simulink model "BatteryEstim3RC_PTBS_estimation"  (R2020b)
settings: Solver=ode45  StartTime=0.0  StopTime=runtime  FixedStep=stepSize  MaxStep=60  RelTol=1e-3
values from neighbouring files (symbols this model uses):
  Q = 277.758    [BatteryEstim3RC_run.m]
undefined symbols (not defined in the file or in its folder): coeff, init_Q, init_Vt, OCV_current, OCV_prev, R0_current, R0_prev, R1_current, R1_prev, R2_current, R2_prev, R3_current, R3_prev, SOC_current, SOC_prev, tau1_current, tau1_prev, tau2_current, tau2_prev, tau3_current, tau3_prev
libraries: autolibbatterycommon x4
settings Model: ModifiedByFormat=The MathWorks, Inc.  Creator=The MathWorks, Inc.  LastModifiedBy=The MathWorks, Inc.
settings DataIOCC: ExternalInput=[input_time input_current]  LoadExternalInput=on  SaveOutput=off  DSMLogging=off  SaveTime=off  ReturnWorkspaceOutputs=off
settings DebuggingCC: ArithmeticOperatorsInVariantConditions=warning
settings SFSimCC: SimUseLocalCustomCode=off  CustomCodeUndefinedFunction=UseInterfaceOnly
settings RTWCC: RTWUseLocalCustomCode=off
settings CodeAppCC: StateflowObjectComments=on

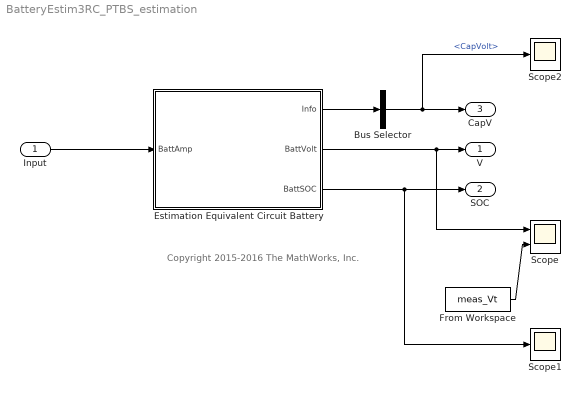
== system BatteryEstim3RC_PTBS_estimation ==
  note: Copyright 2015-2016 The MathWorks, Inc.
  Input : Inport
  Bus Selector : BusSelector  OutputSignals=CapVolt
  Estimation Equivalent Circuit Battery : Subsystem  mask(Estimation Equivalent Circuit Battery){NumRC=3, Em=[OCV_current; OCV_prev], R0=[R0_current; R0_prev], SOC_BP=[SOC_current; SOC_prev], BattCap=Q, BattCapInit=init_Q, InitialCapVoltage=init_Vt, R1=[R1_current; R1_prev], C1=[tau1_current./R1_current; tau1_prev./R1_prev], R2=[R2_current; R2_prev], C2=[tau2_current./R2_current; tau2_prev./R2_prev], R3=[R3_current; R3_prev], C3=[tau3_current./R3_current; tau3_prev./R3_prev], R4=[0.005 0.005 0.005 0.005 0.005 0.005], C4=[10000 10000 10000 10000 10000 10000], R5=[0.005 0.005 0.005 0.005 0.005 0.005], C5=[10000 10000 10000 10000 10000 10000], Vu=Inf, Vl=-Inf}
      mask prompts: NumRC "autoblks:autoblkParamEstRcBattery:blkPrm_NumRC"; Em "autoblks:autoblkParamEstRcBattery:blkPrm_Em"; R0 "autoblks:autoblkParamEstRcBattery:blkPrm_R0"; SOC_BP "autoblks:autoblkParamEstRcBattery:blkPrm_SOC_BP"; BattCap "autoblks:autoblkParamEstRcBattery:blkPrm_BattCap"; BattCapInit "autoblks:autoblkParamEstRcBattery:blkPrm_BattCapInit"; InitialCapVoltage "autoblks:autoblkParamEstRcBattery:blkPrm_InitialCapVoltage"; R1 "autoblks:autoblkParamEstRcBattery:blkPrm_R1"; C1 "autoblks:autoblkParamEstRcBattery:blkPrm_C1"; R2 "autoblks:autoblkParamEstRcBattery:blkPrm_R2"; C2 "autoblks:autoblkParamEstRcBattery:blkPrm_C2"; R3 "autoblks:autoblkParamEstRcBattery:blkPrm_R3"; C3 "autoblks:autoblkParamEstRcBattery:blkPrm_C3"; R4 "autoblks:autoblkParamEstRcBattery:blkPrm_R4"; C4 "autoblks:autoblkParamEstRcBattery:blkPrm_C4"; R5 "autoblks:autoblkParamEstRcBattery:blkPrm_R5"; C5 "autoblks:autoblkParamEstRcBattery:blkPrm_C5"; Vu "autoblks:autoblkParamEstRcBattery:blkPrm_Vu"; Vl "autoblks:autoblkParamEstRcBattery:blkPrm_Vl"
      mask help: autoblks:autoblkParamEstRcBattery:blkDesc
      mask init:
      | autoicon('pbbatteryparamest', gcb, 'Initialization');
      mask Help: eval('autoblkshelp(''pbbatteryrcnetworkpe'')');
      mask TypeOptions NumRC: autoblks:autoblkParamEstRcBattery:blkCmb_NumRC1 | autoblks:autoblkParamEstRcBattery:blkCmb_NumRC2 | autoblks:autoblkParamEstRcBattery:blkCmb_NumRC3 | autoblks:autoblkParamEstRcBattery:blkCmb_NumRC4 | autoblks:autoblkParamEstRcBattery:blkCmb_NumRC5
      mask Callback NumRC: autoicon('pbbatteryparamest', gcb, 'NumRCPopup');
      mask DialogControl Container9 Prompt: autoblks:autoblkParamEstRcBattery:blkDlg_Container9
      mask DialogControl NumRC Prompt: Number of series RC pairs:
      mask DialogControl Em Prompt: Open circuit voltage table data, Em [V]:
      mask DialogControl R0 Prompt: Series resistance table data, R0 [Ohm]:
      mask DialogControl SOC_BP Prompt: State of charge breakpoints, SOC_BP []:
      mask DialogControl BattCap Prompt: Battery capacity, BattCap [Ah]:
      mask DialogControl BattCapInit Prompt: Initial battery capacity, BattCapInit [Ah]:
      mask DialogControl InitialCapVoltage Prompt: Initial capacitor voltage, InitialCapVoltage [V]:
      mask DialogControl Container10 Prompt: autoblks:autoblkParamEstRcBattery:blkDlg_Container10
      mask DialogControl R1 Prompt: Network resistance table data, R1 [Ohm]:
      mask DialogControl C1 Prompt: Network capacitance table data, C1 [F]:
      mask DialogControl R2 Prompt: Network resistance table data, R2 [Ohm]:
      mask DialogControl C2 Prompt: Network capacitance table data, C2 [F]:
      mask DialogControl R3 Prompt: Network resistance table data, R3 [Ohm]:
      mask DialogControl C3 Prompt: Network capacitance table data, C3 [F]:
      mask DialogControl R4 Prompt: Network resistance table data, R4 [Ohm]:
      mask DialogControl C4 Prompt: Network capacitance table data, C4 [F]:
      mask DialogControl R5 Prompt: Network resistance table data, R5 [Ohm]:
      mask DialogControl C5 Prompt: Network capacitance table data, C5 [F]:
      mask DialogControl Container7 Prompt: autoblks:autoblkParamEstRcBattery:blkDlg_Container7
      mask DialogControl Vu Prompt: Upper Integrator Voltage Limit, Vu [V]:
      mask DialogControl Vl Prompt: Lower Integrator Voltage Limit, Vl [V]:
      mask Display:
      | IconInfo = autoicon('pbbatteryparamest', gcb, 'DrawCommands');
      | 
      | image(IconInfo.image, IconInfo.position);
      | 
      | for i = 1:numel(IconInfo.lconn)
      |     port_label('lconn', i, IconInfo.lconn{i})
      | end
      | 
      | for j = 1:numel(IconInfo.rconn)
      |     port_label('rconn', j, IconInfo.rconn{j})
      | end
      | 
      | for k = 1:numel(IconInfo.input)
      |     port_label('input', k, IconInfo.input{k})
      | end
      | 
      | for m = 1:numel(IconInfo.output)
      |     port_label('output', m, IconInfo.output{m})
      | end
  From Workspace : FromWorkspace  VariableName=meas_Vt
  Scope : Scope  NumInputPorts=2
  Scope1 : Scope
  Scope2 : Scope
  V : Outport
  SOC : Outport  Port=2
  CapV : Outport  Port=3
  wires:
  Estimation Equivalent Circuit Battery/1(Info) -> Bus Selector/1
  Bus Selector/1 -> Scope2/1, CapV/1  "<CapVolt>"
  Estimation Equivalent Circuit Battery/3(BattSOC) -> Scope1/1, SOC/1
  Estimation Equivalent Circuit Battery/2(BattVolt) -> Scope/1, V/1
  Input/1 -> Estimation Equivalent Circuit Battery/1(BattAmp)
  From Workspace/1 -> Scope/2

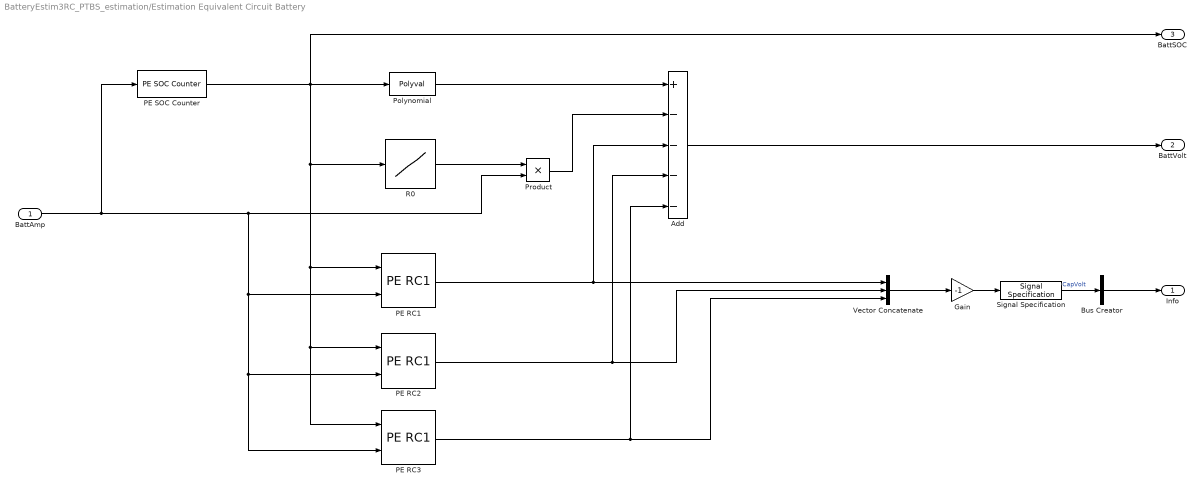
== system BatteryEstim3RC_PTBS_estimation/Estimation Equivalent Circuit Battery ==
  BattAmp : Inport
  Add : Sum  Inputs=+----
  Bus Creator : BusCreator  Inputs=1
  Gain : Gain  Gain=-1
  PE RC1 : autolibbatterycommon/PE RC1  R=R1  C=C1  SOC_BP=SOC_BP  V_init=InitialCapVoltage(1)  V_upper=Vu  V_lower=Vl
      settings: SourceProductBaseCode=PW
  PE RC2 : autolibbatterycommon/PE RC1  R=R2  C=C2  SOC_BP=SOC_BP  V_init=InitialCapVoltage(2)  V_upper=Vu  V_lower=Vl
      settings: SourceProductBaseCode=PW
  PE RC3 : autolibbatterycommon/PE RC1  R=R3  C=C3  SOC_BP=SOC_BP  V_init=InitialCapVoltage(3)  V_upper=Inf  V_lower=-Inf
      settings: SourceProductBaseCode=PW
  PE SOC Counter : autolibbatterycommon/PE SOC Counter  Q_init=BattCapInit  Cap=BattCap
      settings: SourceProductBaseCode=PW
  Polynomial : Polyval  Coefs=coeff
  Product : Product
  R0 : Lookup_n-D  NumberOfTableDimensions=1  LookupTableObject=''  BreakpointsForDimension1=SOC_BP  Table=R0  ExtrapMethod=Clip  UseLastTableValue=on  InternalRulePriority=Speed  RndMeth=Simplest  InputSameDT=on
  Signal Specification : SignalSpecification  Unit=V
  Vector Concatenate : Concatenate  NumInputs=3
  Info : Outport
  BattVolt : Outport  Port=2
  BattSOC : Outport  Port=3
  wires:
  Vector Concatenate/1 -> Gain/1
  PE SOC Counter/1 -> Polynomial/1, BattSOC/1, R0/1, PE RC2/1, PE RC3/1, PE RC1/1
  Polynomial/1 -> Add/1
  PE RC2/1 -> Add/4, Vector Concatenate/2
  PE RC3/1 -> Vector Concatenate/3, Add/5
  PE RC1/1 -> Add/3, Vector Concatenate/1
  Bus Creator/1 -> Info/1
  Gain/1 -> Signal Specification/1
  Add/1 -> BattVolt/1
  Product/1 -> Add/2
  R0/1 -> Product/1
  Signal Specification/1 -> Bus Creator/1  "CapVolt"
  BattAmp/1 -> PE RC2/2, PE RC3/2, PE RC1/2, Product/2, PE SOC Counter/1
